simulink model "example1"  (Simulink 8.2)
settings: Solver=ode45  StartTime=0.0  StopTime=10.0  RelTol=1e-3
settings Model: Creator=Jin  LastModifiedBy=Jin
settings DataIOCC: SignalLoggingSaveFormat=Dataset
settings OptimizationCC: ExpressionDepthLimit=128
settings DebuggingCC: FcnCallInpInsideContextMsg=EnableAllAsError  StateNameClashWarn=none
settings GRTTargetCC: CombineOutputUpdateFcns=on  GRTInterface=off

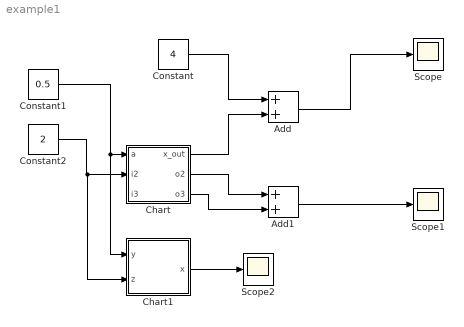
== system example1 ==
  Add : Sum
  Add1 : Sum
  Chart : Stateflow chart  TreatAsAtomicUnit=on
  Chart1 : Stateflow chart  TreatAsAtomicUnit=on
  Constant : Constant  Value=4  OutDataTypeStr=double
  Constant1 : Constant  Value=0.5  OutMin=0  OutMax=3
  Constant2 : Constant  Value=2  OutMin=0  OutMax=3
  Scope : Scope
  Scope1 : Scope
  Scope2 : Scope
      settings: SaveName=ScopeData2
  wires:
  Constant/1 -> Add/1
  Add/1 -> Scope/1
  Chart/1(x_out) -> Add/2
  Constant1/1 -> Chart1/1(y), Chart/1(a)
  Constant2/1 -> Chart1/2(z), Chart/2(i2)
  Chart/2(o2) -> Add1/1
  Chart/3(o3) -> Add1/2
  Add1/1 -> Scope1/1
  Chart1/1(x) -> Scope2/1

== stateflow chart Chart ==
  settings: updateMethod=CONTINUOUS
  state Init
    du:
    x_dot = a;
    x_out = x;
  state Finish
    du:
    x_dot = 0;
    x_out = x;
  (default) -> Init : {x = 1;}
  Init -> Finish : [x >= 7]
  data: x local double; x_out output double =3; a input double; y local double; o2 output double; i2 input double; o3 output double; i3 input double
  data x settings: updateMethod=SF_CONTINUOUS_TIME_DATA

== stateflow chart Chart1 ==
  state Hi
    du:
    x = y + z;
  (default) -> Hi
  data: x output double; y input double; z input double
